simulink model "exercise2"  (R2019b)
settings: Solver=VariableStepAuto  StartTime=0.0  StopTime=10  RelTol=1e-3
settings Model: Creator=adity  LastModifiedBy=adity

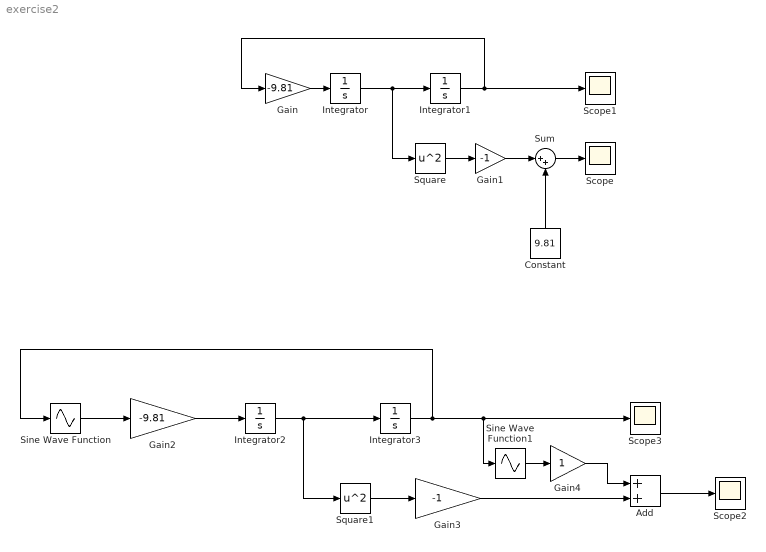
== system exercise2 ==
  Add : Sum
  Constant : Constant  Value=9.81
  Gain : Gain  Gain=-9.81
  Gain1 : Gain  Gain=-1
  Gain2 : Gain  Gain=-9.81
  Gain3 : Gain  Gain=-1
  Gain4 : Gain
  Integrator : Integrator
  Integrator1 : Integrator  InitialCondition=pi/8
  Integrator2 : Integrator
  Integrator3 : Integrator  InitialCondition=pi/8
  Scope{,1..3} (4 alike) : Scope
  Sine Wave Function : Sin  TimeSource=Use external signal  SampleTime=0
  Sine Wave Function1 : Sin  TimeSource=Use external signal  Phase=pi/2  SampleTime=0
  Square : Math  Operator=square  SignedPower=off  SaturateOnIntegerOverflow=on
  Square1 : Math  Operator=square  SignedPower=off  SaturateOnIntegerOverflow=on
  Sum : Sum  Inputs=|++
  wires:
  Gain/1 -> Integrator/1
  Integrator/1 -> Square/1, Integrator1/1
  Constant/1 -> Sum/2
  Gain1/1 -> Sum/1
  Square/1 -> Gain1/1
  Sum/1 -> Scope/1
  Integrator1/1 -> Scope1/1, Gain/1
  Integrator2/1 -> Square1/1, Integrator3/1
  Integrator3/1 -> Scope3/1, Sine Wave Function1/1, Sine Wave Function/1
  Sine Wave Function/1 -> Gain2/1
  Gain2/1 -> Integrator2/1
  Square1/1 -> Gain3/1
  Gain3/1 -> Add/2
  Sine Wave Function1/1 -> Gain4/1
  Gain4/1 -> Add/1
  Add/1 -> Scope2/1
